simulink model "LAB_01_19_SEPT_SIM"  (R2022b)
settings: Solver=VariableStepAuto  StartTime=0.0  StopTime=10.0  RelTol=1e-3
values from neighbouring files (symbols this model uses):
  g = 9.81    [LAB_02_26_SEPT_MAT_PENDULUM.m]
settings Model: Creator=maria  LastModifiedBy=maria
settings OptimizationCC: BlockReduction=off  DefaultParameterBehavior=Inlined  BufferReuse=off

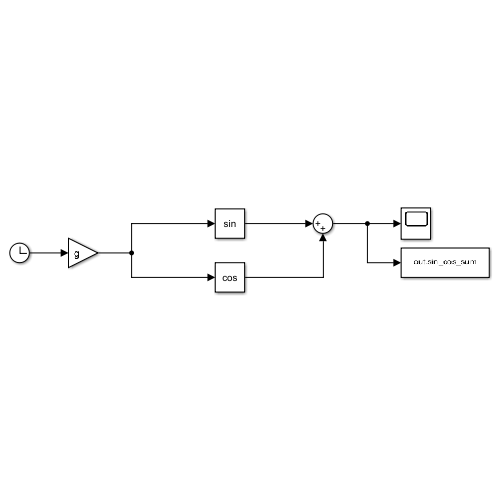
[thumbnail: Simulink's stored preview of the top-level diagram]
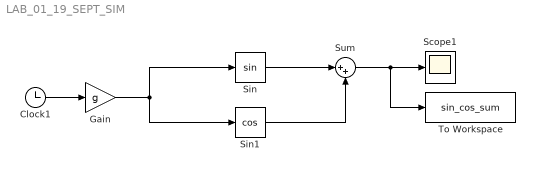
== system LAB_01_19_SEPT_SIM ==
  Clock1 : Clock
  Gain : Gain  Gain=g
  Scope1 : Scope
  Sin : Trigonometry
  Sin1 : Trigonometry  Operator=cos
  Sum : Sum  Inputs=|++
  To Workspace : ToWorkspace  VariableName=sin_cos_sum  SaveFormat=Timeseries  SampleTime=-1
  wires:
  Gain/1 -> Sin1/1, Sin/1
  Sin1/1 -> Sum/2
  Sum/1 -> To Workspace/1, Scope1/1
  Clock1/1 -> Gain/1
  Sin/1 -> Sum/1
